simulink model "Simulink_PID_Cascata"  (R2025b)
settings: Solver=VariableStepAuto  StartTime=0.0  StopTime=30  RelTol=1e-3
InitFcn:
  | run("init.m");
StopFcn:
  | %run("video.m");
values from neighbouring files (symbols this model uses):
  q0_guess = [pi/3; -pi/6; pi/3]    [init.m]
  robot_params = p    [PID.m]    (also in PID_CASCATA.m)
settings Model: Creator=Acer  LastModifiedBy=Acer

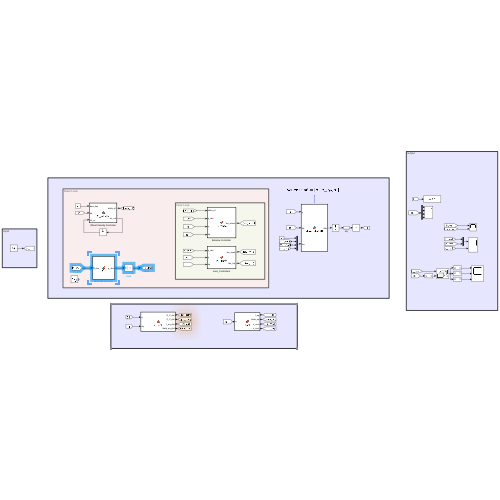
[thumbnail: Simulink's stored preview of the top-level diagram]
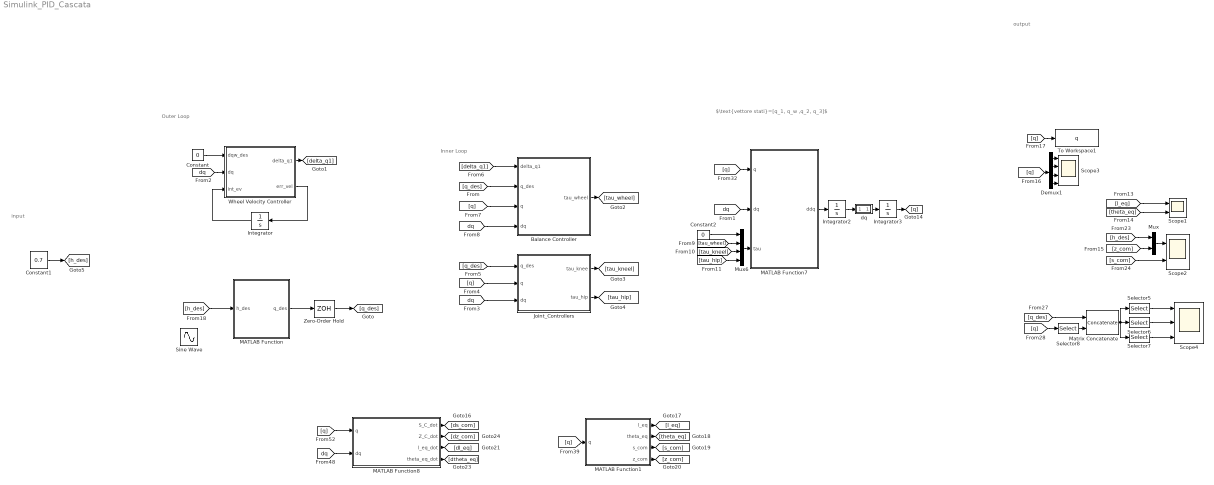
== system Simulink_PID_Cascata ==
  note: input
  note: $\text{vettore stati}=[q_1, q_w ,q_2, q_3]$
  note: Inner Loop
  note: Outer Loop
  note: output
  Balance Controller : MATLAB Function  TreatAsAtomicUnit=on
  Constant : Constant  Value=0
  Constant1 : Constant  Value=0.7
  Constant2 : Constant  Value=0
  Demux1 : Demux
  Integrator : Integrator
  Integrator2 : Integrator  InitialCondition=zeros(4,1)
  Integrator3 : Integrator  InitialCondition=[q0_guess(1);0;q0_guess(2);q0_guess(3)]
  Joint_Controllers : MATLAB Function  TreatAsAtomicUnit=on
  MATLAB Function : MATLAB Function  TreatAsAtomicUnit=on
  MATLAB Function1 : MATLAB Function  TreatAsAtomicUnit=on
  MATLAB Function7 : MATLAB Function  TreatAsAtomicUnit=on
  MATLAB Function8 : MATLAB Function  TreatAsAtomicUnit=on
  Matrix Concatenate : Concatenate  Mode=Multidimensional array  ConcatenateDimension=2
  Mux : Mux  Inputs=2
  Mux6 : Mux
  Scope1 : Scope  NumInputPorts=2
      settings: ActiveDisplayYMinimum=0.018273571358949733  ActiveDisplayYMaximum=1.1017296672248229
  Scope2 : Scope  NumInputPorts=2
      settings: ActiveDisplayYMinimum=-0.80168815443654451  ActiveDisplayYMaximum=0.86685423938183825  DataLoggingVariableName=ScopeData2
  Scope3 : Scope  NumInputPorts=4
      settings: ActiveDisplayYMinimum=0.39796467970383342  ActiveDisplayYMaximum=6.8902933946314784  DataLoggingVariableName=ScopeData4
  Scope4 : Scope  NumInputPorts=3
      settings: ActiveDisplayYMinimum=-1.6006235510725582  ActiveDisplayYMaximum=3.15753292524381  DataLoggingVariableName=ScopeData3
  Selector5 : Selector  NumberOfDimensions=2  InputPortWidth=3  IndexOptions=Index vector (dialog),Index vector (dialog)  Indices=[1],[1 2]  OutputSizes=1,1
  Selector6 : Selector  NumberOfDimensions=2  InputPortWidth=3  IndexOptions=Index vector (dialog),Index vector (dialog)  Indices=[2],[1 2]  OutputSizes=1,1
  Selector7 : Selector  NumberOfDimensions=2  InputPortWidth=3  IndexOptions=Index vector (dialog),Index vector (dialog)  Indices=[3],[1 2]  OutputSizes=1,1
  Selector8 : Selector  InputPortWidth=4  IndexOptions=Index vector (dialog)  Indices=[1 3 4]  OutputSizes=1
  Sine Wave : Sin  Amplitude=0.1  Bias=0.7  SampleTime=0
  To Workspace1 : ToWorkspace  VariableName=q  SaveFormat=Timeseries  SampleTime=-1
  Wheel Velocity Controller : MATLAB Function  TreatAsAtomicUnit=on
  Zero-Order Hold : ZeroOrderHold  SampleTime=-1
  dq : Subsystem
  wires:
  Mux6/1 -> MATLAB Function7/3(tau)
  [q] -> MATLAB Function7/1(q)
  Integrator3/1 -> [q]
  MATLAB Function7/1(ddq) -> Integrator2/1
  [dq] -> MATLAB Function7/2(dq)
  Constant/1 -> Wheel Velocity Controller/1(dqw_des)
  [dq] -> Wheel Velocity Controller/2(dq)
  Integrator2/1 -> dq/1(In1)
  dq/1(Out1) -> Integrator3/1
  [dq] -> Joint_Controllers/3(dq)
  [q] -> Joint_Controllers/2(q)
  [q_des] -> Balance Controller/2(q_des)
  [q_des] -> Joint_Controllers/1(q_des)
  Wheel Velocity Controller/1(delta_q1) -> [delta_q1]
  [delta_q1] -> Balance Controller/1(delta_q1)
  [q] -> Balance Controller/3(q)
  [dq] -> Balance Controller/4(dq)
  Wheel Velocity Controller/2(err_vel) -> Integrator/1
  Integrator/1 -> Wheel Velocity Controller/3(int_ev)
  MATLAB Function/1(q_des) -> Zero-Order Hold/1
  Balance Controller/1(tau_wheel) -> [tau_wheel]
  Joint_Controllers/1(tau_knee) -> [tau_kneel]
  Joint_Controllers/2(tau_hip) -> [tau_hip]
  [tau_wheel] -> Mux6/2
  [tau_kneel] -> Mux6/3
  [tau_hip] -> Mux6/4
  Constant2/1 -> Mux6/1
  Zero-Order Hold/1 -> [q_des]
  Mux/1 -> Scope2/1
  [s_com] -> Scope2/2
  [h_des] -> Mux/1
  [z_com] -> Mux/2
  [theta_eq] -> Scope1/2
  [l_eq] -> Scope1/1
  MATLAB Function8/1(S_C_dot) -> [ds_com]
  [dq] -> MATLAB Function8/2(dq)
  MATLAB Function8/3(l_eq_dot) -> [dl_eq]
  MATLAB Function1/2(theta_eq) -> [theta_eq]
  [q] -> MATLAB Function1/1(q)
  [q] -> MATLAB Function8/1(q)
  MATLAB Function1/1(l_eq) -> [l_eq]
  MATLAB Function8/4(theta_eq_dot) -> [dtheta_eq]
  MATLAB Function1/3(s_com) -> [s_com]
  MATLAB Function8/2(Z_C_dot) -> [dz_com]
  MATLAB Function1/4(z_com) -> [z_com]
  Selector8/1 -> Matrix Concatenate/2
  [q] -> Selector8/1
  Selector7/1 -> Scope4/3
  Selector6/1 -> Scope4/2
  Selector5/1 -> Scope4/1
  Matrix Concatenate/1 -> Selector6/1, Selector5/1, Selector7/1
  [q_des] -> Matrix Concatenate/1
  [q] -> To Workspace1/1
  [q] -> Demux1/1
  Demux1/4 -> Scope3/4
  Demux1/3 -> Scope3/3
  Demux1/1 -> Scope3/1
  Demux1/2 -> Scope3/2
  Constant1/1 -> [h_des]
  [h_des] -> MATLAB Function/1(h_des)

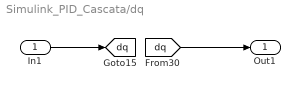
== system Simulink_PID_Cascata/dq ==
  In1 : Inport
  Out1 : Outport
  tag scope: dq=global
  wires:
  In1/1 -> [dq]
  [dq] -> Out1/1

== matlab function Simulink_PID_Cascata/Balance Controller ==
  data: delta_q1 input; tau_wheel output; q_des input; q input; dq input
function tau_wheel = PD_Wheel(delta_q1, q_des, q, dq)

% Il target reale dello stinco è ora modificato dal loop di velocità!
    q1_target_new = q_des(1) + delta_q1; 
    
    Kp_w = 400;  % Guadagno proporzionale ruota
    Kd_w = 80;   % Guadagno derivativo ruota
    
    e1 = q1_target_new - q(1);
    de1 = 0 - dq(1);
    
    % Generazione coppia di bilanciamento
    tau_wheel = Kp_w * e1 + Kd_w * de1;

== matlab function Simulink_PID_Cascata/Wheel Velocity Controller ==
  data: dqw_des input; delta_q1 output; dq input; int_ev input; err_vel output
function [delta_q1, err_vel] = PI_Velocity(dqw_des, dq, int_ev)

    % dqw_des velocita di riferimento della ruota
    
    err_vel = dqw_des - dq(2); % Errore di velocità della ruota
    
    % Guadagni PI (relativamente piccoli perché mappano velocità in radianti di inclinazione)
    Kp_v = 0.08; 
    Ki_v = 0.06;

    % L'output del loop di velocità è un "Angle Offset" (delta_q1)
    delta_q1 = -(Kp_v * err_vel + Ki_v * int_ev);

    % Saturazione di sicurezza per evitare che l'offset richieda inclinazioni estreme
    delta_q1 = max(min(delta_q1, 0.2), -0.2);

== matlab function Simulink_PID_Cascata/Joint_Controllers ==
  data: q_des input; tau_knee output; q input; tau_hip output; dq input
function [tau_knee, tau_hip] = PD_Joints(q_des, q, dq)

    Kp_j = 800; 
    Kd_j = 50;  
    
    e2 = q_des(2) - q(3);
    de2 = 0 - dq(3);
    tau_knee = Kp_j * e2 + Kd_j * de2;
    
    e3 = q_des(3) - q(4);
    de3 = 0 - dq(4);
    tau_hip = Kp_j * e3 + Kd_j * de3;

== matlab function Simulink_PID_Cascata/MATLAB Function ==
  settings: updateMethod=DISCRETE  sampleTime=0.1
  data: h_des input; q_des output; robot_params parameter; q0_guess parameter
function q_des = fcn(h_des, robot_params, q0_guess)
    % 1. Pre-allocazione per dire a Simulink che uscirà un vettore 3x1
    q_des = zeros(3,1);
    
    % 2. Dichiara la TUA funzione esterna come estrinseca (non fsolve)
    coder.extrinsic('calcola_target_cinematici');
    
    % 3. Inizializza la variabile temporanea per aiutare il Coder con i tipi
    q_des_calc = zeros(3,1);
    
    % 4. Richiama la funzione (il calcolo viene "appaltato" a MATLAB)
    q_des_calc = calcola_target_cinematici(h_des, robot_params, q0_guess);
    
    % 5. Assegnazione sicura all'uscita
    if ~isempty(q_des_calc)
        q_des = q_des_calc;
    end
end

== matlab function Simulink_PID_Cascata/MATLAB Function1 ==
  data: q input size=4; l_eq output; theta_eq output; s_com output; z_com output; robot_params parameter
function [l_eq,theta_eq, s_com, z_com] = CoM(q,robot_params)

[l_eq,theta_eq, s_com, z_com] = calcola_CoM_equivalente(q, robot_params);

end

== matlab function Simulink_PID_Cascata/MATLAB Function7 ==
  data: q input; ddq output size=4; dq input; tau input
function ddq =  whole_robot_2D(q, dq, tau)
    % tau è il vettore delle coppie/forze generalizzate in ingresso (4x1)
    
    [M, CdQ, G] = calc_dynamics(q, dq);

    %% equazione del moto: M*ddq + C*dq + G = tau
    % In MATLAB/Simulink si usa l'operatore mldivide (\) per invertire M in modo robusto
    ddq = M \ (tau - CdQ - G);
end

== matlab function Simulink_PID_Cascata/MATLAB Function8 ==
  data: q input; dq input; S_C_dot output; Z_C_dot output; l_eq_dot output; theta_eq_dot output; robot_params parameter
function [S_C_dot, Z_C_dot, l_eq_dot, theta_eq_dot] = J_CoM(q,dq,robot_params)
    %#codegen
    % CALCOLA_VELOCITA_COM_SIMULINK Calcola le velocità del CoM e del pendolo 
    % equivalente (WIP) per l'utilizzo in Simulink.
    
    % --- 1. Estrazione Variabili di Stato ---
    q1 = q(1);
    q2 = q(3);
    q3 = q(4);
    
    % --- 2. Estrazione Parametri Robot ---
    l1 = robot_params.l1;
    l2 = robot_params.l2;
    l3 = robot_params.l3;
    
    m1 = robot_params.m1;
    m2 = robot_params.m2;
    m3 = robot_params.m3;
    m_upper = m1 + m2 + m3;
    
    % --- 3. Costanti Raggruppate per l'Analitica ---
    K1 = (m1 * (l1/2) + m2 * l1 + m3 * l1) / m_upper;
    K2 = (m2 * (l2/2) + m3 * l2) / m_upper;
    K3 = (m3 * (l3/2)) / m_upper;
    
    % --- 4. Ricalcolo Posizione CoM ---
    S_C = K1*cos(q1) + K2*cos(q1+q2) + K3*sin(q3);
    Z_C = K1*sin(q1) + K2*sin(q1+q2) + K3*cos(q3);
    
    % --- 5. Calcolo Jacobiano (J_CoM) ---
    % Preallocazione statica della matrice 2x4 per compatibilità C/C++
    J_CoM = zeros(2, 4);
    
    % Derivate parziali di S_C (Prima Riga)
    J_CoM(1, 2) = -K1*sin(q1) - K2*sin(q1+q2);
    J_CoM(1, 3) = -K2*sin(q1+q2);
    J_CoM(1, 4) =  K3*cos(q3);
    
    % Derivate parziali di Z_C (Seconda Riga)
    J_CoM(2, 2) =  K1*cos(q1) + K2*cos(q1+q2);
    J_CoM(2, 3) =  K2*cos(q1+q2);
    J_CoM(2, 4) = -K3*sin(q3);
    
    % --- 6. Calcolo Velocità Cartesiane ---
    % V_C = [S_C_dot; Z_C_dot]
    V_C = J_CoM * dq;
    S_C_dot = V_C(1);
    Z_C_dot = V_C(2);
    
    % --- 7. Derivate del Pendolo Equivalente e Gestione Singolarità ---
    l_eq_sq = S_C^2 + Z_C^2;
    l_eq = sqrt(l_eq_sq);
    

        l_eq_dot = (S_C * S_C_dot + Z_C * Z_C_dot) / l_eq;
        theta_eq_dot = (S_C_dot * Z_C - S_C * Z_C_dot) / l_eq_sq;
   end
